simulink model "inverted_pendulum"  (R2017a)
settings: Solver=FixedStepAuto  StartTime=0.0  StopTime=20  FixedStep=0.01  RelTol=1e-3
undefined symbols (not defined in the file): gamma, Jt, k1, k1_, k2, k2_, l1, l2, len, mg, omega0, omega1, theta0, theta1
settings Model: Creator=tonypai  LastModifiedBy=tonypai

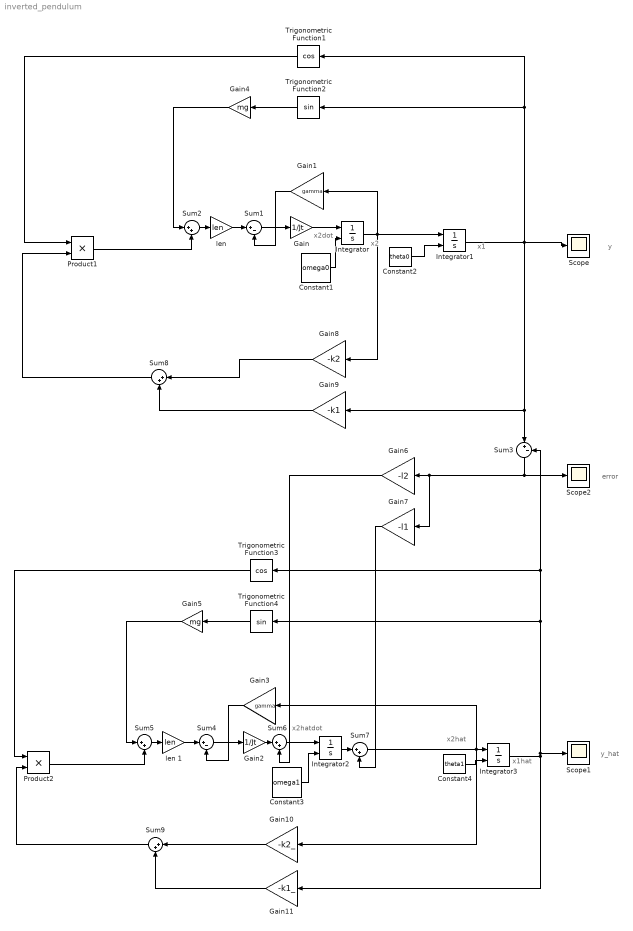
== system inverted_pendulum ==
  note: y
  note: x2dot
  note: x2
  note: x1
  note: y_hat
  note: error
  note: x2hat
  note: x1hat
  note: x2hatdot
  Constant1 : Constant  Value=omega0
  Constant2 : Constant  Value=theta0
  Constant3 : Constant  Value=omega1
  Constant4 : Constant  Value=theta1
  Gain : Gain  Gain=1/Jt
  Gain1 : Gain  Gain=gamma
  Gain10 : Gain  Gain=-k2_
  Gain11 : Gain  Gain=-k1_
  Gain2 : Gain  Gain=1/Jt
  Gain3 : Gain  Gain=gamma
  Gain4 : Gain  Gain=mg
  Gain5 : Gain  Gain=mg
  Gain6 : Gain  Gain=-l2
  Gain7 : Gain  Gain=-l1
  Gain8 : Gain  Gain=-k2
  Gain9 : Gain  Gain=-k1
  Integrator{,1..3} (4 alike) : Integrator  InitialConditionSource=external
  Product1 : Product
  Product2 : Product
  Scope : Scope
  Scope1 : Scope
  Scope2 : Scope
  Sum1 : Sum  Inputs=|+-
  Sum{2,5..9} (6 alike) : Sum  Inputs=|++
  Sum3 : Sum  Inputs=|+-
  Sum4 : Sum  Inputs=|+-
  Trigonometric Function1 : Trigonometry  Operator=cos
  Trigonometric Function2 : Trigonometry
  Trigonometric Function3 : Trigonometry  Operator=cos
  Trigonometric Function4 : Trigonometry
  "len " : Gain  Gain=len
  len 1 : Gain  Gain=len
  wires:
  Trigonometric Function2/1 -> Gain4/1
  Gain4/1 -> Sum2/1
  "len "/1 -> Sum1/1
  Gain1/1 -> Sum1/2
  Sum1/1 -> Gain/1
  Gain/1 -> Integrator/1
  Constant1/1 -> Integrator/2
  Constant2/1 -> Integrator1/2
  Integrator/1 -> Gain8/1, Integrator1/1, Gain1/1
  Sum2/1 -> "len "/1
  Trigonometric Function1/1 -> Product1/1
  Product1/1 -> Sum2/2
  Sum8/1 -> Product1/2
  Integrator1/1 -> Gain9/1, Sum3/1, Scope/1, Trigonometric Function2/1, Trigonometric Function1/1
  Constant3/1 -> Integrator2/2
  Sum4/1 -> Gain2/1
  Trigonometric Function4/1 -> Gain5/1
  len 1/1 -> Sum4/1
  Constant4/1 -> Integrator3/2
  Trigonometric Function3/1 -> Product2/1
  Sum3/1 -> Gain7/1, Gain6/1, Scope2/1
  Product2/1 -> Sum5/2
  Sum5/1 -> len 1/1
  Gain3/1 -> Sum4/2
  Gain5/1 -> Sum5/1
  Gain8/1 -> Sum8/1
  Gain9/1 -> Sum8/2
  Gain11/1 -> Sum9/2
  Gain10/1 -> Sum9/1
  Sum9/1 -> Product2/2
  Integrator3/1 -> Gain11/1, Trigonometric Function4/1, Trigonometric Function3/1, Sum3/2, Scope1/1
  Gain2/1 -> Sum6/1
  Gain6/1 -> Sum6/2
  Sum6/1 -> Integrator2/1
  Integrator2/1 -> Sum7/1
  Gain7/1 -> Sum7/2
  Sum7/1 -> Gain10/1, Gain3/1, Integrator3/1
